simulink model "Zone_1_Zone_2_Thyristor_240Hz"  (R2025b)
settings: Solver=FixedStepDiscrete  StartTime=0.0  StopTime=5  FixedStep=Ts  RelTol=1e-3  EnableMultiTasking=on
undefined symbols (not defined in the file or in its folder): DiscIntNeverNeededParam, GABDA, GABDB, GBBDA, GBBDB, GPPMA, GPPMB, GPPMC, SADA, SADB, SADC, SADD, SBDA, SBDB, SBDC, SCDA, SCDB, SCDC, SCDD, SDDA, SDDB, SDDC, SDDD, SDDE, Ts, TsELEC
libraries: nesl_utility x70, fl_lib x60, ee_lib x44, eeThyristorSixPulseGenerator x2, eePowerMeasurement x2, eeSinusoidalMeasurement x2
(part 1 of 3)
settings Model: Creator=gdudgeon  LastModifiedBy=gdudgeon
settings SolverCC: ConcurrentTasks=on  AlgebraicLoopSolver=TrustRegion  AutoInsertRateTranBlk=on
settings DataIOCC: SaveFormat=StructureWithTime  SaveOutput=off  SignalLogging=off  DSMLogging=off  SaveTime=off
settings OptimizationCC: BlockReduction=off  OptimizeBlockIOStorage=off  BufferReuse=off  GlobalBufferReuse=off  ExpressionFolding=off  LocalBlockOutputs=off  OptimizeDataStoreBuffers=off  BusAssignmentInplaceUpdate=off
settings DebuggingCC: UnconnectedInputMsg=warning  UnconnectedOutputMsg=warning  UnconnectedLineMsg=warning
settings HardwareCC: ProdBitPerPointer=32.0  ProdBitPerSizeT=32.0  ProdBitPerPtrDiffT=32.0  ProdLargestAtomicFloat=None  ProdWordSize=32.0  ProdLongLongMode=on  ProdHWDeviceType=Generic->32-bit x86 compatible
settings ModelReferenceCC: EnableRefExpFcnMdlSchedulingChecks=on  ModelReferenceNumInstancesAllowed=Single  ModelReferenceMinAlgLoopOccurrences=on
settings SFSimCC: CustomCodeUndefinedFunction=UseInterfaceOnly
settings RTWCC: SystemTargetFile=slrt.tlc  TLCOptions=-axPCMaxOverloads=3000  TemplateMakefile=slrt_default_tmf  CodeProfilingInstrumentation=coarse  RTWCompilerOptimization=on  GPUComputeCapability=3.5  Description=Simulink Real-Time
settings SimulinkRealTimeCC: RL32LogTETModifier=off  xPCConcurrentTasks=on  MultiwordLength=2048.0  DynamicStringBufferSize=256.0  PreserveMATLABNamespacesInGeneratedCode=on  SubcomponentCodeInterfacePackaging=Nonreusable function  SupportVariableSizeSignals=on  InstructionSetFMA=off  OptimizeReductions=off  LogToMDFFile=off

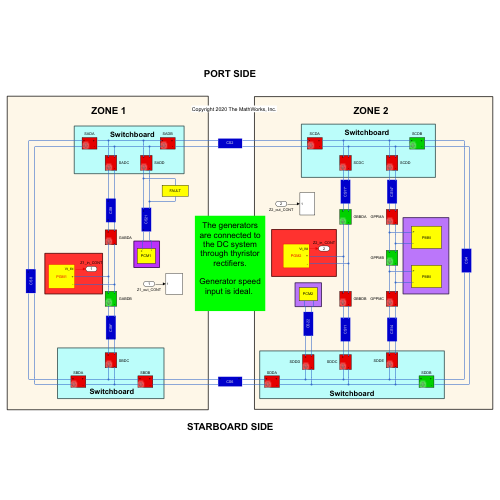
[thumbnail: Simulink's stored preview of the top-level diagram]
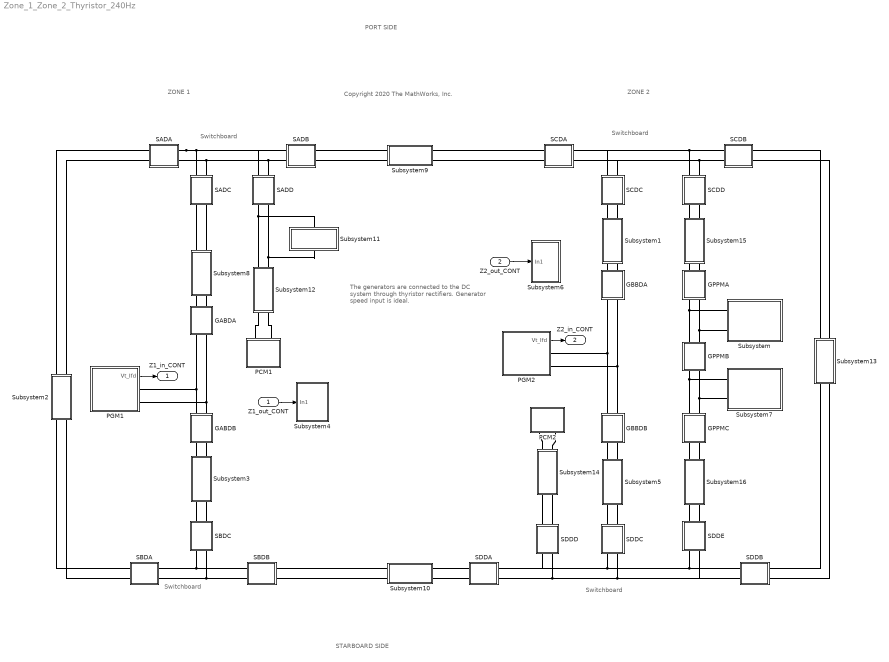
== system Zone_1_Zone_2_Thyristor_240Hz ==
  note: Copyright 2020 The MathWorks, Inc.
  note: The generators are connected to the DC system through thyristor rectifiers.
      |
      | Generator speed input is ideal.
  note: Switchboard
  note: Switchboard
  note: Switchboard
  note: ZONE 1
  note: Switchboard
  note: ZONE 2
  note: PORT SIDE
  note: STARBOARD SIDE
  Z1_out_CONT : Inport  OutDataTypeStr=double  PortDimensions=11
  Z2_out_CONT : Inport  Port=2  OutDataTypeStr=double  PortDimensions=17
  GABDA : Subsystem  mask{status=GABDA}
      mask prompts: status "Initial Status"
      mask init:
      | if ~status
      |     
      |     set(gcbh,'BackgroundColor','green')
      |     
      | elseif status
      |     
      |     set(gcbh,'BackgroundColor','red')
      |     
      | end
  GABDB : Subsystem  mask{status=GABDB}
      mask prompts: status "Initial Status"
      mask init:
      | if ~status
      |     
      |     set(gcbh,'BackgroundColor','green')
      |     
      | elseif status
      |     
      |     set(gcbh,'BackgroundColor','red')
      |     
      | end
  GBBDA : Subsystem  mask{status=GBBDA}
      mask prompts: status "Initial Status"
      mask init:
      | if ~status
      |     
      |     set(gcbh,'BackgroundColor','green')
      |     
      | elseif status
      |     
      |     set(gcbh,'BackgroundColor','red')
      |     
      | end
  GBBDB : Subsystem  mask{status=GBBDB}
      mask prompts: status "Initial Status"
      mask init:
      | if ~status
      |     
      |     set(gcbh,'BackgroundColor','green')
      |     
      | elseif status
      |     
      |     set(gcbh,'BackgroundColor','red')
      |     
      | end
  GPPMA : Subsystem  mask{status=GPPMA}
      mask prompts: status "Initial Status"
      mask init:
      | if ~status
      |     
      |     set(gcbh,'BackgroundColor','green')
      |     
      | elseif status
      |     
      |     set(gcbh,'BackgroundColor','red')
      |     
      | end
  GPPMB : Subsystem  mask{status=GPPMB}
      mask prompts: status "Initial Status"
      mask init:
      | if ~status
      |     
      |     set(gcbh,'BackgroundColor','green')
      |     
      | elseif status
      |     
      |     set(gcbh,'BackgroundColor','red')
      |     
      | end
  GPPMC : Subsystem  mask{status=GPPMC}
      mask prompts: status "Initial Status"
      mask init:
      | if ~status
      |     
      |     set(gcbh,'BackgroundColor','green')
      |     
      | elseif status
      |     
      |     set(gcbh,'BackgroundColor','red')
      |     
      | end
  PCM1 : Subsystem
      mask Display: disp('PCM1')
  PCM2 : Subsystem
      mask Display: disp('PCM2')
  PGM1 : Subsystem
      mask Display: disp('PGM1')
  PGM2 : Subsystem
      mask Display: disp('PGM2')
  SADA : Subsystem  mask{status=SADA}
      mask prompts: status "Initial Status"
      mask init:
      | if ~status
      |     
      |     set(gcbh,'BackgroundColor','green')
      |     
      | elseif status
      |     
      |     set(gcbh,'BackgroundColor','red')
      |     
      | end
  SADB : Subsystem  mask{status=SADB}
      mask prompts: status "Initial Status"
      mask init:
      | if ~status
      |     
      |     set(gcbh,'BackgroundColor','green')
      |     
      | elseif status
      |     
      |     set(gcbh,'BackgroundColor','red')
      |     
      | end
  SADC : Subsystem  mask{status=SADC}
      mask prompts: status "Initial Status"
      mask init:
      | if ~status
      |     
      |     set(gcbh,'BackgroundColor','green')
      |     
      | elseif status
      |     
      |     set(gcbh,'BackgroundColor','red')
      |     
      | end
  SADD : Subsystem  mask{status=SADD}
      mask prompts: status "Initial Status"
      mask init:
      | if ~status
      |     
      |     set(gcbh,'BackgroundColor','green')
      |     
      | elseif status
      |     
      |     set(gcbh,'BackgroundColor','red')
      |     
      | end
  SBDA : Subsystem  mask{status=SBDA}
      mask prompts: status "Initial Status"
      mask init:
      | if ~status
      |     
      |     set(gcbh,'BackgroundColor','green')
      |     
      | elseif status
      |     
      |     set(gcbh,'BackgroundColor','red')
      |     
      | end
  SBDB : Subsystem  mask{status=SBDB}
      mask prompts: status "Initial Status"
      mask init:
      | if ~status
      |     
      |     set(gcbh,'BackgroundColor','green')
      |     
      | elseif status
      |     
      |     set(gcbh,'BackgroundColor','red')
      |     
      | end
  SBDC : Subsystem  mask{status=SBDC}
      mask prompts: status "Initial Status"
      mask init:
      | if ~status
      |     
      |     set(gcbh,'BackgroundColor','green')
      |     
      | elseif status
      |     
      |     set(gcbh,'BackgroundColor','red')
      |     
      | end
  SCDA : Subsystem  mask{status=SCDA}
      mask prompts: status "Initial Status"
      mask init:
      | if ~status
      |     
      |     set(gcbh,'BackgroundColor','green')
      |     
      | elseif status
      |     
      |     set(gcbh,'BackgroundColor','red')
      |     
      | end
  SCDB : Subsystem  mask{status=SCDB}
      mask prompts: status "Initial Status"
      mask init:
      | if ~status
      |     
      |     set(gcbh,'BackgroundColor','green')
      |     
      | elseif status
      |     
      |     set(gcbh,'BackgroundColor','red')
      |     
      | end
  SCDC : Subsystem  mask{status=SCDC}
      mask prompts: status "Initial Status"
      mask init:
      | if ~status
      |     
      |     set(gcbh,'BackgroundColor','green')
      |     
      | elseif status
      |     
      |     set(gcbh,'BackgroundColor','red')
      |     
      | end
  SCDD : Subsystem  mask{status=SCDD}
      mask prompts: status "Initial Status"
      mask init:
      | if ~status
      |     
      |     set(gcbh,'BackgroundColor','green')
      |     
      | elseif status
      |     
      |     set(gcbh,'BackgroundColor','red')
      |     
      | end
  SDDA : Subsystem  mask{status=SDDA}
      mask prompts: status "Initial Status"
      mask init:
      | if ~status
      |     
      |     set(gcbh,'BackgroundColor','green')
      |     
      | elseif status
      |     
      |     set(gcbh,'BackgroundColor','red')
      |     
      | end
  SDDB : Subsystem  mask{status=SDDB}
      mask prompts: status "Initial Status"
      mask init:
      | if ~status
      |     
      |     set(gcbh,'BackgroundColor','green')
      |     
      | elseif status
      |     
      |     set(gcbh,'BackgroundColor','red')
      |     
      | end
  SDDC : Subsystem  mask{status=SDDC}
      mask prompts: status "Initial Status"
      mask init:
      | if ~status
      |     
      |     set(gcbh,'BackgroundColor','green')
      |     
      | elseif status
      |     
      |     set(gcbh,'BackgroundColor','red')
      |     
      | end
  SDDD : Subsystem  mask{status=SDDD}
      mask prompts: status "Initial Status"
      mask init:
      | if ~status
      |     
      |     set(gcbh,'BackgroundColor','green')
      |     
      | elseif status
      |     
      |     set(gcbh,'BackgroundColor','red')
      |     
      | end
  SDDE : Subsystem  mask{status=SDDE}
      mask prompts: status "Initial Status"
      mask init:
      | if ~status
      |     
      |     set(gcbh,'BackgroundColor','green')
      |     
      | elseif status
      |     
      |     set(gcbh,'BackgroundColor','red')
      |     
      | end
  Subsystem : Subsystem
      mask Display: disp('PMM')
  Subsystem1 : Subsystem
      mask Display: disp('CS11*')
  Subsystem10 : Subsystem
      mask Display: disp('CS6')
  Subsystem11 : Subsystem
      mask Display: disp('FAULT')
  Subsystem12 : Subsystem
      mask Display: disp('CS21')
  Subsystem13 : Subsystem
      mask Display: disp('CS4')
  Subsystem14 : Subsystem
      mask Display: disp('CS22')
  Subsystem15 : Subsystem
      mask Display: disp('CS14*')
  Subsystem16 : Subsystem
      mask Display: disp('CS14')
  Subsystem2 : Subsystem
      mask Display: disp('CS8')
  Subsystem3 : Subsystem
      mask Display: disp('CS9*')
  Subsystem4 : Subsystem
  Subsystem5 : Subsystem
      mask Display: disp('CS11')
  Subsystem6 : Subsystem
  Subsystem7 : Subsystem
      mask Display: disp('PMM')
  Subsystem8 : Subsystem
      mask Display: disp('CS9')
  Subsystem9 : Subsystem
      mask Display: disp('CS2')
  Z1_in_CONT : Outport  OutDataTypeStr=double  PortDimensions=2
  Z2_in_CONT : Outport  Port=2  OutDataTypeStr=double  PortDimensions=2
  wires:
  PGM2/1(Vt_Ifd) -> Z2_in_CONT/1
  PGM1/1(Vt_Ifd) -> Z1_in_CONT/1
  Z1_out_CONT/1 -> Subsystem4/1(In1)
  Z2_out_CONT/1 -> Subsystem6/1(In1)
  connections:
  GBBDA/RConn1 -- PGM2/RConn1 -- GBBDB/LConn1
  SDDB/LConn2 -- SDDE/RConn2 -- SDDC/RConn2 -- SDDD/RConn2 -- SDDA/RConn2
  SDDD/RConn1 -- SDDA/RConn1 -- SDDC/RConn1 -- SDDB/LConn1 -- SDDE/RConn1
  GBBDB/LConn2 -- PGM2/RConn2 -- GBBDA/RConn2
  Subsystem16/RConn2 -- SDDE/LConn2
  GBBDB/RConn1 -- Subsystem5/LConn1
  Subsystem16/RConn1 -- SDDE/LConn1
  SDDC/LConn1 -- Subsystem5/RConn1
  SDDC/LConn2 -- Subsystem5/RConn2
  Subsystem10/LConn1 -- SDDA/LConn1
  GBBDB/RConn2 -- Subsystem5/LConn2
  Subsystem10/LConn2 -- SDDA/LConn2
  SCDD/LConn2 -- SCDB/LConn2 -- SCDA/RConn2 -- SCDC/LConn2
  SCDD/LConn1 -- SCDB/LConn1 -- SCDA/RConn1 -- SCDC/LConn1
  Subsystem15/LConn1 -- SCDD/RConn1
  Subsystem15/LConn2 -- SCDD/RConn2
  GBBDA/LConn2 -- Subsystem1/RConn2
  GBBDA/LConn1 -- Subsystem1/RConn1
  SCDC/RConn1 -- Subsystem1/LConn1
  SCDC/RConn2 -- Subsystem1/LConn2
  Subsystem13/LConn1 -- SCDB/RConn1
  SCDB/RConn2 -- Subsystem13/LConn2
  Subsystem13/RConn1 -- SDDB/RConn1
  SDDB/RConn2 -- Subsystem13/RConn2
  SADA/RConn2 -- SADB/LConn2 -- SADD/LConn2 -- SADC/LConn2
  SBDC/RConn2 -- SBDA/RConn2 -- SBDB/LConn2
  GABDB/LConn2 -- PGM1/RConn2 -- GABDA/RConn2
  GABDB/LConn1 -- PGM1/RConn1 -- GABDA/RConn1
  SADA/RConn1 -- SADC/LConn1 -- SADB/LConn1 -- SADD/LConn1
  SBDC/RConn1 -- SBDA/RConn1 -- SBDB/LConn1
  GABDB/RConn1 -- Subsystem3/LConn1
  GABDA/LConn2 -- Subsystem8/RConn2
  GABDA/LConn1 -- Subsystem8/RConn1
  SBDA/LConn1 -- Subsystem2/RConn1
  Subsystem2/LConn2 -- SADA/LConn2
  SADC/RConn2 -- Subsystem8/LConn2
  SADC/RConn1 -- Subsystem8/LConn1
  Subsystem10/RConn2 -- SBDB/RConn2
  Subsystem2/LConn1 -- SADA/LConn1
  GABDB/RConn2 -- Subsystem3/LConn2
  SBDC/LConn2 -- Subsystem3/RConn2
  Subsystem10/RConn1 -- SBDB/RConn1
  SBDC/LConn1 -- Subsystem3/RConn1
  SBDA/LConn2 -- Subsystem2/RConn2
  Subsystem9/RConn1 -- SADB/RConn1
  Subsystem9/RConn2 -- SADB/RConn2
  SCDA/LConn1 -- Subsystem9/LConn1
  Subsystem9/LConn2 -- SCDA/LConn2
  Subsystem12/RConn2 -- PCM1/LConn2
  Subsystem12/RConn1 -- PCM1/LConn1
  Subsystem12/LConn1 -- Subsystem11/LConn1 -- SADD/RConn1
  SADD/RConn2 -- Subsystem11/RConn1 -- Subsystem12/LConn2
  Subsystem14/LConn1 -- PCM2/LConn1
  PCM2/LConn2 -- Subsystem14/LConn2
  Subsystem14/RConn1 -- SDDD/LConn1
  SDDD/LConn2 -- Subsystem14/RConn2
  GPPMC/RConn2 -- Subsystem16/LConn2
  GPPMC/RConn1 -- Subsystem16/LConn1
  GPPMA/LConn1 -- Subsystem15/RConn1
  GPPMA/LConn2 -- Subsystem15/RConn2
  GPPMA/RConn1 -- Subsystem/LConn1 -- GPPMB/LConn1
  GPPMA/RConn2 -- Subsystem/LConn2 -- GPPMB/LConn2
  GPPMB/RConn1 -- Subsystem7/LConn1 -- GPPMC/LConn1
  GPPMB/RConn2 -- Subsystem7/LConn2 -- GPPMC/LConn2

== system Zone_1_Zone_2_Thyristor_240Hz/GABDA ==
  SADC : ee_lib/Switches & Breakers/DPST Switch  R_closed=1e-3 Ohm  G_open=1e-6 S  Threshold=0.5 V  Width=0 V  model_dynamics=0  t_on=1e-3 s  t_off=1e-3 s  initial_vT=0 V
      settings: InternalSimscapePortConfiguration="{\"Bottom\":[],\"Left\":[{\"id\":\"vT\",\"label\":\"vT\",\"type\":\"input\"},{\"id\":\"p1\",\"label\":\"\",\"type\":\"foundation.electrical.electrical\"},{\"id\":\"p2\",\"label\":\"\",\"type\":\"foundation.electrical.electrical\"}],\"Right\":[{\"id\":\"n1\",\"label\":\"\",\"type\":\"foundation.electrical.electrical\"},{\"id\":\"n2\",\"label\":\"\",\"type\":\"foundation.electrical.electrical\"}],\"Top\":[]}"
  Simulink-PS Converter : nesl_utility/Simulink-PS Converter  PhysicalDomain=network_engine_domain  SubClassName=ps_input  LeftPortType=input  RightPortType=output  PseudoPeriodic=off  Frequencies=[]  NoiseDistribution=none  NoiseParameters=[]  Unit=1  AffineConversion=off  FilteringAndDerivatives=provide  SimscapeFilterOrder=1  InputFilterTimeConstant=0.001  UdotUserProvided=0
  "+ " : PMIOPort  Side=Right
  + : PMIOPort  Port=2  Side=Left
  "- " : PMIOPort  Port=3  Side=Right
  - : PMIOPort  Port=4  Side=Left
  wires:
  [GABDA] -> Simulink-PS Converter/1  "GABDA"
  connections:
  Simulink-PS Converter/RConn1 -- SADC/LConn1
  SADC/LConn2 -- +/RConn1
  SADC/LConn3 -- -/RConn1
  SADC/RConn2 -- "- "/RConn1
  SADC/RConn1 -- "+ "/RConn1

== system Zone_1_Zone_2_Thyristor_240Hz/GABDB ==
  GABDB : ee_lib/Switches & Breakers/DPST Switch  R_closed=1e-3 Ohm  G_open=1e-6 S  Threshold=0.5 V  Width=0 V  model_dynamics=0  t_on=1e-3 s  t_off=1e-3 s  initial_vT=0 V
      settings: InternalSimscapePortConfiguration="{\"Bottom\":[],\"Left\":[{\"id\":\"vT\",\"label\":\"vT\",\"type\":\"input\"},{\"id\":\"p1\",\"label\":\"\",\"type\":\"foundation.electrical.electrical\"},{\"id\":\"p2\",\"label\":\"\",\"type\":\"foundation.electrical.electrical\"}],\"Right\":[{\"id\":\"n1\",\"label\":\"\",\"type\":\"foundation.electrical.electrical\"},{\"id\":\"n2\",\"label\":\"\",\"type\":\"foundation.electrical.electrical\"}],\"Top\":[]}"
  Simulink-PS Converter : nesl_utility/Simulink-PS Converter  PhysicalDomain=network_engine_domain  SubClassName=ps_input  LeftPortType=input  RightPortType=output  PseudoPeriodic=off  Frequencies=[]  NoiseDistribution=none  NoiseParameters=[]  Unit=1  AffineConversion=off  FilteringAndDerivatives=provide  SimscapeFilterOrder=1  InputFilterTimeConstant=0.001  UdotUserProvided=0
  "+ " : PMIOPort  Side=Right
  + : PMIOPort  Port=2  Side=Left
  "- " : PMIOPort  Port=3  Side=Right
  - : PMIOPort  Port=4  Side=Left
  wires:
  [GABDB] -> Simulink-PS Converter/1
  connections:
  GABDB/RConn1 -- "+ "/RConn1
  GABDB/LConn3 -- -/RConn1
  GABDB/RConn2 -- "- "/RConn1
  Simulink-PS Converter/RConn1 -- GABDB/LConn1
  GABDB/LConn2 -- +/RConn1

== system Zone_1_Zone_2_Thyristor_240Hz/GBBDA ==
  SADC : ee_lib/Switches & Breakers/DPST Switch  R_closed=1e-3 Ohm  G_open=1e-6 S  Threshold=0.5 V  Width=0 V  model_dynamics=0  t_on=1e-3 s  t_off=1e-3 s  initial_vT=0 V
      settings: InternalSimscapePortConfiguration="{\"Bottom\":[],\"Left\":[{\"id\":\"vT\",\"label\":\"vT\",\"type\":\"input\"},{\"id\":\"p1\",\"label\":\"\",\"type\":\"foundation.electrical.electrical\"},{\"id\":\"p2\",\"label\":\"\",\"type\":\"foundation.electrical.electrical\"}],\"Right\":[{\"id\":\"n1\",\"label\":\"\",\"type\":\"foundation.electrical.electrical\"},{\"id\":\"n2\",\"label\":\"\",\"type\":\"foundation.electrical.electrical\"}],\"Top\":[]}"
  Simulink-PS Converter : nesl_utility/Simulink-PS Converter  PhysicalDomain=network_engine_domain  SubClassName=ps_input  LeftPortType=input  RightPortType=output  PseudoPeriodic=off  Frequencies=[]  NoiseDistribution=none  NoiseParameters=[]  Unit=1  AffineConversion=off  FilteringAndDerivatives=provide  SimscapeFilterOrder=1  InputFilterTimeConstant=0.001  UdotUserProvided=0
  "+ " : PMIOPort  Side=Right
  + : PMIOPort  Port=2  Side=Left
  "- " : PMIOPort  Port=3  Side=Right
  - : PMIOPort  Port=4  Side=Left
  wires:
  [GBBDA] -> Simulink-PS Converter/1
  connections:
  SADC/LConn1 -- Simulink-PS Converter/RConn1
  SADC/RConn1 -- "+ "/RConn1
  SADC/RConn2 -- "- "/RConn1
  SADC/LConn2 -- +/RConn1
  SADC/LConn3 -- -/RConn1

== system Zone_1_Zone_2_Thyristor_240Hz/GBBDB ==
  GBBDB : ee_lib/Switches & Breakers/DPST Switch  R_closed=1e-3 Ohm  G_open=1e-6 S  Threshold=0.5 V  Width=0 V  model_dynamics=0  t_on=1e-3 s  t_off=1e-3 s  initial_vT=0 V
      settings: InternalSimscapePortConfiguration="{\"Bottom\":[],\"Left\":[{\"id\":\"vT\",\"label\":\"vT\",\"type\":\"input\"},{\"id\":\"p1\",\"label\":\"\",\"type\":\"foundation.electrical.electrical\"},{\"id\":\"p2\",\"label\":\"\",\"type\":\"foundation.electrical.electrical\"}],\"Right\":[{\"id\":\"n1\",\"label\":\"\",\"type\":\"foundation.electrical.electrical\"},{\"id\":\"n2\",\"label\":\"\",\"type\":\"foundation.electrical.electrical\"}],\"Top\":[]}"
  Simulink-PS Converter : nesl_utility/Simulink-PS Converter  PhysicalDomain=network_engine_domain  SubClassName=ps_input  LeftPortType=input  RightPortType=output  PseudoPeriodic=off  Frequencies=[]  NoiseDistribution=none  NoiseParameters=[]  Unit=1  AffineConversion=off  FilteringAndDerivatives=provide  SimscapeFilterOrder=1  InputFilterTimeConstant=0.001  UdotUserProvided=0
  "+ " : PMIOPort  Side=Right
  + : PMIOPort  Port=2  Side=Left
  "- " : PMIOPort  Port=3  Side=Right
  - : PMIOPort  Port=4  Side=Left
  wires:
  [GBBDB] -> Simulink-PS Converter/1
  connections:
  GBBDB/RConn1 -- "+ "/RConn1
  GBBDB/LConn3 -- -/RConn1
  GBBDB/RConn2 -- "- "/RConn1
  Simulink-PS Converter/RConn1 -- GBBDB/LConn1
  GBBDB/LConn2 -- +/RConn1

== system Zone_1_Zone_2_Thyristor_240Hz/GPPMA ==
  SADC : ee_lib/Switches & Breakers/DPST Switch  R_closed=1e-3 Ohm  G_open=1e-6 S  Threshold=0.5 V  Width=0 V  model_dynamics=0  t_on=1e-3 s  t_off=1e-3 s  initial_vT=0 V
      settings: InternalSimscapePortConfiguration="{\"Bottom\":[],\"Left\":[{\"id\":\"vT\",\"label\":\"vT\",\"type\":\"input\"},{\"id\":\"p1\",\"label\":\"\",\"type\":\"foundation.electrical.electrical\"},{\"id\":\"p2\",\"label\":\"\",\"type\":\"foundation.electrical.electrical\"}],\"Right\":[{\"id\":\"n1\",\"label\":\"\",\"type\":\"foundation.electrical.electrical\"},{\"id\":\"n2\",\"label\":\"\",\"type\":\"foundation.electrical.electrical\"}],\"Top\":[]}"
  Simulink-PS Converter : nesl_utility/Simulink-PS Converter  PhysicalDomain=network_engine_domain  SubClassName=ps_input  LeftPortType=input  RightPortType=output  PseudoPeriodic=off  Frequencies=[]  NoiseDistribution=none  NoiseParameters=[]  Unit=1  AffineConversion=off  FilteringAndDerivatives=provide  SimscapeFilterOrder=1  InputFilterTimeConstant=0.001  UdotUserProvided=0
  "+ " : PMIOPort  Side=Right
  + : PMIOPort  Port=2  Side=Left
  "- " : PMIOPort  Port=3  Side=Right
  - : PMIOPort  Port=4  Side=Left
  wires:
  [GPPMA] -> Simulink-PS Converter/1
  connections:
  SADC/RConn2 -- "- "/RConn1
  SADC/RConn1 -- "+ "/RConn1
  SADC/LConn2 -- +/RConn1
  SADC/LConn3 -- -/RConn1
  Simulink-PS Converter/RConn1 -- SADC/LConn1

== system Zone_1_Zone_2_Thyristor_240Hz/GPPMB ==
  SADC : ee_lib/Switches & Breakers/DPST Switch  R_closed=1e-3 Ohm  G_open=1e-6 S  Threshold=0.5 V  Width=0 V  model_dynamics=0  t_on=1e-3 s  t_off=1e-3 s  initial_vT=0 V
      settings: InternalSimscapePortConfiguration="{\"Bottom\":[],\"Left\":[{\"id\":\"vT\",\"label\":\"vT\",\"type\":\"input\"},{\"id\":\"p1\",\"label\":\"\",\"type\":\"foundation.electrical.electrical\"},{\"id\":\"p2\",\"label\":\"\",\"type\":\"foundation.electrical.electrical\"}],\"Right\":[{\"id\":\"n1\",\"label\":\"\",\"type\":\"foundation.electrical.electrical\"},{\"id\":\"n2\",\"label\":\"\",\"type\":\"foundation.electrical.electrical\"}],\"Top\":[]}"
  Simulink-PS Converter : nesl_utility/Simulink-PS Converter  PhysicalDomain=network_engine_domain  SubClassName=ps_input  LeftPortType=input  RightPortType=output  PseudoPeriodic=off  Frequencies=[]  NoiseDistribution=none  NoiseParameters=[]  Unit=1  AffineConversion=off  FilteringAndDerivatives=provide  SimscapeFilterOrder=1  InputFilterTimeConstant=0.001  UdotUserProvided=0
  "+ " : PMIOPort  Side=Right
  + : PMIOPort  Port=2  Side=Left
  "- " : PMIOPort  Port=3  Side=Right
  - : PMIOPort  Port=4  Side=Left
  wires:
  [GPPMB] -> Simulink-PS Converter/1
  connections:
  Simulink-PS Converter/RConn1 -- SADC/LConn1
  SADC/LConn3 -- -/RConn1
  SADC/LConn2 -- +/RConn1
  SADC/RConn1 -- "+ "/RConn1
  SADC/RConn2 -- "- "/RConn1

== system Zone_1_Zone_2_Thyristor_240Hz/GPPMC ==
  SADC : ee_lib/Switches & Breakers/DPST Switch  R_closed=1e-3 Ohm  G_open=1e-6 S  Threshold=0.5 V  Width=0 V  model_dynamics=0  t_on=1e-3 s  t_off=1e-3 s  initial_vT=0 V
      settings: InternalSimscapePortConfiguration="{\"Bottom\":[],\"Left\":[{\"id\":\"vT\",\"label\":\"vT\",\"type\":\"input\"},{\"id\":\"p1\",\"label\":\"\",\"type\":\"foundation.electrical.electrical\"},{\"id\":\"p2\",\"label\":\"\",\"type\":\"foundation.electrical.electrical\"}],\"Right\":[{\"id\":\"n1\",\"label\":\"\",\"type\":\"foundation.electrical.electrical\"},{\"id\":\"n2\",\"label\":\"\",\"type\":\"foundation.electrical.electrical\"}],\"Top\":[]}"
  Simulink-PS Converter : nesl_utility/Simulink-PS Converter  PhysicalDomain=network_engine_domain  SubClassName=ps_input  LeftPortType=input  RightPortType=output  PseudoPeriodic=off  Frequencies=[]  NoiseDistribution=none  NoiseParameters=[]  Unit=1  AffineConversion=off  FilteringAndDerivatives=provide  SimscapeFilterOrder=1  InputFilterTimeConstant=0.001  UdotUserProvided=0
  "+ " : PMIOPort  Side=Right
  + : PMIOPort  Port=2  Side=Left
  "- " : PMIOPort  Port=3  Side=Right
  - : PMIOPort  Port=4  Side=Left
  wires:
  [GPPMC] -> Simulink-PS Converter/1
  connections:
  SADC/RConn2 -- "- "/RConn1
  SADC/RConn1 -- "+ "/RConn1
  SADC/LConn2 -- +/RConn1
  SADC/LConn3 -- -/RConn1
  Simulink-PS Converter/RConn1 -- SADC/LConn1

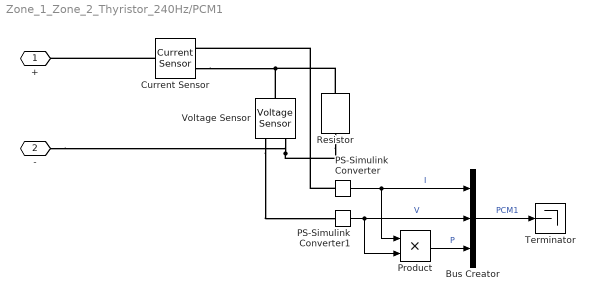
== system Zone_1_Zone_2_Thyristor_240Hz/PCM1 ==
  Bus Creator : BusCreator  Inputs=3
  Current Sensor : fl_lib/Electrical/Electrical Sensors/Current Sensor
  PS-Simulink Converter : nesl_utility/PS-Simulink Converter  PhysicalDomain=network_engine_domain  SubClassName=ps_output  LeftPortType=input  RightPortType=output  PseudoPeriodic=off  Frequencies=[]  VectorFormat=1-D array  Unit=1  AffineConversion=off
  PS-Simulink Converter1 : nesl_utility/PS-Simulink Converter  PhysicalDomain=network_engine_domain  SubClassName=ps_output  LeftPortType=input  RightPortType=output  PseudoPeriodic=off  Frequencies=[]  VectorFormat=1-D array  Unit=1  AffineConversion=off
  Product : Product
  Resistor : fl_lib/Electrical/Electrical Elements/Resistor  R=20 Ohm  i_specify=off  i_priority=None  i=0 A  i_nominal_specify=off  i_nominal_value=1  i_nominal_unit=A  v_specify=off  v_priority=None  v=0 V  v_nominal_specify=off  v_nominal_value=1  v_nominal_unit=V
  Terminator : Terminator
  Voltage Sensor : fl_lib/Electrical/Electrical Sensors/Voltage Sensor
  + : PMIOPort  Side=Left
  - : PMIOPort  Port=2  Side=Left
  wires:
  PS-Simulink Converter/1 -> Product/1, Bus Creator/1  "I"
  PS-Simulink Converter1/1 -> Product/2, Bus Creator/2  "V"
  Product/1 -> Bus Creator/3  "P"
  Bus Creator/1 -> Terminator/1  "PCM1"
  connections:
  Current Sensor/RConn2 -- Resistor/LConn1 -- Voltage Sensor/LConn1
  Voltage Sensor/RConn2 -- -/RConn1 -- Resistor/RConn1
  PS-Simulink Converter/LConn1 -- Current Sensor/RConn1
  Voltage Sensor/RConn1 -- PS-Simulink Converter1/LConn1
  Current Sensor/LConn1 -- +/RConn1

== system Zone_1_Zone_2_Thyristor_240Hz/PCM2 ==
  Bus Creator : BusCreator  Inputs=3
  Current Sensor : fl_lib/Electrical/Electrical Sensors/Current Sensor
  PS-Simulink Converter : nesl_utility/PS-Simulink Converter  PhysicalDomain=network_engine_domain  SubClassName=ps_output  LeftPortType=input  RightPortType=output  PseudoPeriodic=off  Frequencies=[]  VectorFormat=1-D array  Unit=1  AffineConversion=off
  PS-Simulink Converter1 : nesl_utility/PS-Simulink Converter  PhysicalDomain=network_engine_domain  SubClassName=ps_output  LeftPortType=input  RightPortType=output  PseudoPeriodic=off  Frequencies=[]  VectorFormat=1-D array  Unit=1  AffineConversion=off
  Product : Product
  Resistor : fl_lib/Electrical/Electrical Elements/Resistor  R=100 Ohm  i_specify=off  i_priority=None  i=0 A  i_nominal_specify=off  i_nominal_value=1  i_nominal_unit=A  v_specify=off  v_priority=None  v=0 V  v_nominal_specify=off  v_nominal_value=1  v_nominal_unit=V
  Terminator : Terminator
  Voltage Sensor : fl_lib/Electrical/Electrical Sensors/Voltage Sensor
  + : PMIOPort  Side=Left
  - : PMIOPort  Port=2  Side=Left
  wires:
  PS-Simulink Converter/1 -> Product/1, Bus Creator/1  "I"
  PS-Simulink Converter1/1 -> Product/2, Bus Creator/2  "V"
  Product/1 -> Bus Creator/3  "P"
  Bus Creator/1 -> Terminator/1  "PCM2"
  connections:
  Current Sensor/RConn2 -- Resistor/LConn1 -- Voltage Sensor/LConn1
  Voltage Sensor/RConn2 -- -/RConn1 -- Resistor/RConn1
  PS-Simulink Converter/LConn1 -- Current Sensor/RConn1
  Voltage Sensor/RConn1 -- PS-Simulink Converter1/LConn1
  +/RConn1 -- Current Sensor/LConn1

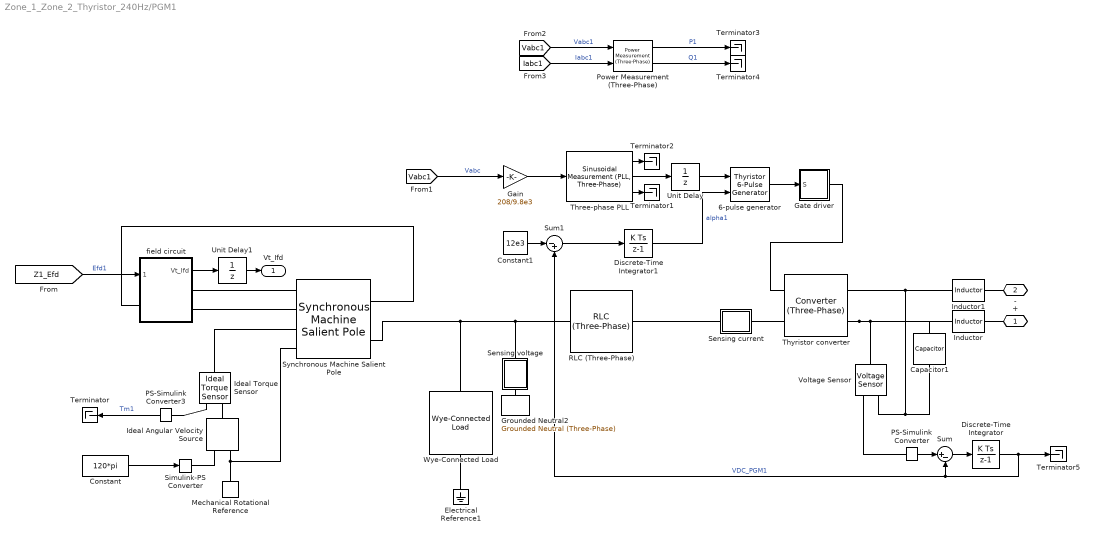
== system Zone_1_Zone_2_Thyristor_240Hz/PGM1 ==
  " field circuit" : Subsystem
  6-pulse generator : eeThyristorSixPulseGenerator/Thyristor 6-Pulse Generator  Ord=Sequential device order  Pw=5*pi/6  Ts=TsELEC
  Capacitor1 : fl_lib/Electrical/Electrical Elements/Capacitor  c=835e-6 F  r=0.075 Ohm  g=0 1/Ohm  i_specify=off  i_priority=None  i=0 A  i_nominal_specify=off  i_nominal_value=1  i_nominal_unit=A  v_specify=on  v_priority=None  v=12e3 V  v_nominal_specify=off  v_nominal_value=1  v_nominal_unit=V  vc_specify=on  vc_priority=High  vc=12e3 V  vc_nominal_specify=off  vc_nominal_value=1  vc_nominal_unit=V
  Constant : Constant  Value=120*pi  SampleTime=TsELEC
  Constant1 : Constant  Value=12e3
  Discrete-Time Integrator : DiscreteIntegrator  gainval=100  InitialCondition=12e3  SampleTime=TsELEC  ICPrevOutput=DiscIntNeverNeededParam  ICPrevScaledInput=DiscIntNeverNeededParam
  Discrete-Time Integrator1 : DiscreteIntegrator  gainval=0.01  InitialCondition=0.9  SampleTime=TsELEC  LimitOutput=on  LowerSaturationLimit=0  ICPrevOutput=DiscIntNeverNeededParam  ICPrevScaledInput=DiscIntNeverNeededParam
  Electrical Reference1 : fl_lib/Electrical/Electrical Elements/Electrical Reference
  Gain : Gain  Gain=208/9.8e3
  Gate driver : Subsystem
  Grounded Neutral2 : ee_lib/Connectors & References/Grounded Neutral (Three-Phase)
  Ideal Angular Velocity Source : fl_lib/Mechanical/Mechanical Sources/Ideal Angular Velocity Source
  Ideal Torque Sensor : fl_lib/Mechanical/Mechanical Sensors/Ideal Torque Sensor
  Inductor : fl_lib/Electrical/Electrical Elements/Inductor  l=790e-6/2 H  r=0.075/2 Ohm  g=1e-9 1/Ohm  i_specify=off  i_priority=None  i=0 A  i_nominal_specify=off  i_nominal_value=1  i_nominal_unit=A  v_specify=off  v_priority=None  v=0 V  v_nominal_specify=off  v_nominal_value=1  v_nominal_unit=V  i_L_specify=off  i_L_priority=High  i_L=0 A  i_L_nominal_specify=off  i_L_nominal_value=1  i_L_nominal_unit=A
  Inductor1 : fl_lib/Electrical/Electrical Elements/Inductor  l=790e-6/2 H  r=0.075/2 Ohm  g=1e-9 1/Ohm  i_specify=off  i_priority=None  i=0 A  i_nominal_specify=off  i_nominal_value=1  i_nominal_unit=A  v_specify=off  v_priority=None  v=0 V  v_nominal_specify=off  v_nominal_value=1  v_nominal_unit=V  i_L_specify=off  i_L_priority=High  i_L=0 A  i_L_nominal_specify=off  i_L_nominal_value=1  i_L_nominal_unit=A
  Mechanical Rotational Reference : fl_lib/Mechanical/Rotational Elements/Mechanical Rotational Reference
  PS-Simulink Converter : nesl_utility/PS-Simulink Converter  PhysicalDomain=network_engine_domain  SubClassName=ps_output  LeftPortType=input  RightPortType=output  PseudoPeriodic=off  Frequencies=[]  VectorFormat=1-D array  Unit=inherit  AffineConversion=off
  PS-Simulink Converter3 : nesl_utility/PS-Simulink Converter  PhysicalDomain=network_engine_domain  SubClassName=ps_output  LeftPortType=input  RightPortType=output  PseudoPeriodic=off  Frequencies=[]  VectorFormat=1-D array  Unit=inherit  AffineConversion=off
  Power Measurement (Three-Phase) : eePowerMeasurement/Power Measurement (Three-Phase)  LabelModeActiveChoice=Discrete  F=60  K=[0 1 2 3]  Seq=Positive  Ts=Ts
  RLC (Three-Phase) : ee_lib/Passive/RLC Assemblies/RLC (Three-Phase)  port_option=ee.enum.threePhasePort.composite  component_structure=2  R=1 Ohm  L=5e-4 H  C=1e-6 F  R_parasitic=1e-6 Ohm  G_parasitic=1e-6 1/Ohm  IL_specify=on  IL_priority=High  IL=[0, 0, 0] A  IL_nominal_specify=off  IL_nominal_value=1  IL_nominal_unit=A  VC_specify=on  VC_priority=High  VC=[0, 0, 0] V  VC_nominal_specify=off  VC_nominal_value=1  VC_nominal_unit=V
      settings: InternalSimscapePortConfiguration="{\"Bottom\":[],\"Left\":[{\"id\":\"N1\",\"label\":\"~1\",\"type\":\"foundation.electrical.three_phase\"}],\"Right\":[{\"id\":\"N2\",\"label\":\"~2\",\"type\":\"foundation.electrical.three_phase\"}],\"Top\":[]}"
  Sensing current : Subsystem
      mask Display: disp('i')
  Sensing voltage : Subsystem
  Simulink-PS Converter : nesl_utility/Simulink-PS Converter  PhysicalDomain=network_engine_domain  SubClassName=ps_input  LeftPortType=input  RightPortType=output  PseudoPeriodic=off  Frequencies=[]  NoiseDistribution=none  NoiseParameters=[]  Unit=rad/s  AffineConversion=off  FilteringAndDerivatives=provide  SimscapeFilterOrder=1  InputFilterTimeConstant=0.001  UdotUserProvided=0
  Sum : Sum  Inputs=|+-
  Sum1 : Sum  Inputs=|-+
  Synchronous Machine Salient Pole : ee_lib/Electromechanical/Synchronous/Synchronous Machine Salient Pole  port_option=ee.enum.threePhasePort.composite  SRated=45e6 V*A  VRated=9.8e3 V  FRated=240 Hz  nPolePairs=4  param_option=ee.enum.sm.parameterization.standard  fieldCircuitParameterization_option=ee.enum.sm.fieldparameterization.current  baseEfd=216.54 V  baseIfd=200 A  zero_sequence=ee.enum.park.zerosequence.exclude  axes_param=ee.enum.rotorangle.daxis  Ladu=0.9  Laqu=0.55  L0=0.15  Ll=0.15  Ra=0.006  Lfd=0.2571  Rfd=0.0006  L1d=0.2  R1d=0.0354  L1q=0.2567  R1q=0.0428  Xl=0.08  Xd=1.352  Xq=0.836  X0=0.15  Xdd=0.296  Xddd=0.148  Xqdd=0.122  d_option=ee.enum.circuit.open  Td0d=4.141 s  Tdd=1.75 s  Td0dd=0.027 s  Tddd=0.0214 s  q_option=ee.enum.circuit.open  Tq0dd=0.184 s  Tqdd=0.0232 s  saturation_option=ee.enum.saturation.exclude  saturation_ifd=[0, .48, .76, 1.38, 1.79]  saturation_Vag=[0, .43, .59, .71, .76]  initialization_option=ee.enum.sm.initialization.electrical  source_type=ee.enum.sm.load_flow_source_type.Swing  Vmag0=13.8e3 V  Vang0=0 deg  Pt0=1e6 V*A  Qt0=0 V*A  minimum_pu=0.95  phase_search_range=[-30, 30] deg  gmin=1e-6 S  connection_option=ee.enum.Connection.wye  num_q_dampers=1  rotor_offset=-pi / 2 rad  pu_psid_specify=off  pu_psid_priority=None  pu_psid=0  pu_psid_nominal_specify=off  pu_psid_nominal_value=1  pu_psid_nominal_unit=1  pu_psiq_specify=off  pu_psiq_priority=None  pu_psiq=0  pu_psiq_nominal_specify=off  pu_psiq_nominal_value=1  pu_psiq_nominal_unit=1  pu_psifd_specify=off  pu_psifd_priority=None  pu_psifd=0  pu_psifd_nominal_specify=off  pu_psifd_nominal_value=1  pu_psifd_nominal_unit=1  pu_psi1d_specify=off  pu_psi1d_priority=None  pu_psi1d=0  pu_psi1d_nominal_specify=off  pu_psi1d_nominal_value=1  pu_psi1d_nominal_unit=1  pu_psi1q_specify=off  pu_psi1q_priority=None  pu_psi1q=0  pu_psi1q_nominal_specify=off  pu_psi1q_nominal_value=1  pu_psi1q_nominal_unit=1  angular_position_diff_specify=off  angular_position_diff_priority=None  angular_position_diff=18 deg  angular_position_diff_nominal_specify=off  angular_position_diff_nominal_value=1  angular_position_diff_nominal_unit=deg  Tmeas=298.15 K  alpha=3.93e-3 1/K  stator_thermal_mass=100 J/K  rotor_thermal_mass=200 J/K  temperatureA_specify=off  temperatureA_priority=High  temperatureA=25 degC  temperatureA_nominal_specify=off  temperatureA_nominal_value=1  temperatureA_nominal_unit=degC  temperatureB_specify=off  temperatureB_priority=High  temperatureB=25 degC  temperatureB_nominal_specify=off  temperatureB_nominal_value=1  temperatureB_nominal_unit=degC  temperatureC_specify=off  temperatureC_priority=High  temperatureC=25 degC  temperatureC_nominal_specify=off  temperatureC_nominal_value=1  temperatureC_nominal_unit=degC  temperatureR_specify=off  temperatureR_priority=High  temperatureR=25 degC  temperatureR_nominal_specify=off  temperatureR_nominal_value=1  temperatureR_nominal_unit=degC
      settings: InternalSimscapePortConfiguration="{\"Bottom\":[],\"Left\":[{\"id\":\"fd_p\",\"label\":\"fd+\",\"type\":\"foundation.electrical.electrical\"},{\"id\":\"fd_n\",\"label\":\"fd-\",\"type\":\"foundation.electrical.electrical\"},{\"id\":\"R\",\"label\":\"R\",\"type\":\"foundation.mechanical.rotational.rotational\"},{\"id\":\"C\",\"label\":\"C\",\"type\":\"foundation.mechanical.rotational.rotational\"}],\"Right\":[{\"id\":\"pu_output\",\"label\":\"pu\",\"type\":\"output\"},{\"id\":\"N\",\"label\":\"~\",\"type\":\"foundation.electrical.three_phase\"}],\"Top\":[]}"
  Terminator{,1..5} (6 alike) : Terminator
  Three-phase PLL : eeSinusoidalMeasurement/Sinusoidal Measurement (PLL, Three-Phase)  Kp_LF=45  Ki_LF=1250  F0=60  Theta0=0  Ts=TsELEC
  Thyristor converter : ee_lib/Semiconductors & Converters/Converters/Converter (Three-Phase)  port_option=ee.enum.threePhasePort.composite  fidelity_option=ee.enum.converters.fidelity.detailed  device_type=ee.enum.converters.switchingdevice.thyristor  showThermalPort=false  K=0  Vth=6 V  Vgt=.5 V  Vgt_off=-1 V  Ih=1 A  Vf=0.8 V  Ron=0.001 Ohm  Rds=0.001 Ohm  Goff=1e-5 1/Ohm  Eon_scalar=22.86e-3 J  Eoff_scalar=17.14e-3 J  Eoff_natural_commutation=10e-3 J  Voff=300 V  Iout_scalar=600 A  onCurrentMeasDelay=0 s  useCurrentFromPreviousCycle=false  useVoltageFromPreviousCycle=false  diode_param=ee.enum.converters.protectiondiode.none  diode_Vf=0.8 V  diode_Ron=0.001 Ohm  diode_Goff=1e-5 1/Ohm  diode_C=50 nF  diode_iRM=-235 A  diode_iF=300 A  diode_idot=-50 A/us  diode_trr_param=ee.enum.converters.diodetrr.trr_factor  diode_trr_factor=3  diode_trr=15 us  diode_Qrr=1.5e+3 s*uA  diode_rec_loss_model=ee.enum.diode.reverseRecoveryModel.fixed  diode_ErecVal=0 J  diode_scaleWithIandV=false  diode_ErecMat=zeros(2, 3) J  diode_TjrecVec=[298.15, 398.15] K  diode_IfrecVec=[.1, 1, 10] A  diode_IrecVal=10 A  diode_VrecVal=10 V  diode_tFilter=1 / 1000 / 100 s  thermal_network_parameterization=ee.enum.thermalNetworkTopology.external  Rth=[.08, .5] K/W  Rth_Cauer=[.08, .1, .5] K/W  Rth_Foster=[.08, .14, .22, .16] K/W  thermal_mass_parameterization=ee.enum.thermalNetwork.timeconstant  thermal_mass=[.01, .5] J/K  thermal_mass_Cauer=[.01, .1, .5] J/K  thermal_mass_Foster=[.001, .005, .05, .5] J/K  thermal_time_constant=[.001, .2] s  thermal_time_constant_Cauer=[.001, .1, .2] s  thermal_time_constant_Foster=[7e-05, .0007, .01, .08] s  thermal_mass_initial_temperatures=[25, 25] degC  thermal_mass_initial_temperatures_Cauer=[25, 25, 25] degC  junction_thermal_mass=0.01 J/K  Tvec_initial_Foster=[25, 25, 25, 25] degC  snubber_type=ee.enum.converters.snubber.exclude  Cs=1e-7 F  Rs=0.1 Ohm  Vce_loss=[0, 150, 300] V
  Unit Delay : UnitDelay  SampleTime=TsELEC  HasFrameUpgradeWarning=on
  Unit Delay1 : UnitDelay  SampleTime=-1  HasFrameUpgradeWarning=on
  Voltage Sensor : fl_lib/Electrical/Electrical Sensors/Voltage Sensor
  Wye-Connected Load : ee_lib/Passive/RLC Assemblies/Wye-Connected Load  port_option=ee.enum.threePhasePort.composite  parameterization=2  component_structure=1  component_structure_PQ=1  R=1 Ohm  L=1e-3 H  C=1e-6 F  VRated=9.8e3 V  FRated=60 Hz  P=1.8e6 W  Qpos=1e2 V*A  Qneg=-1e2 V*A  R_parasitic=1e-6 Ohm  G_parasitic=1e-6 1/Ohm  R_parasitic_PQ=1e-6 Ohm  G_parasitic_PQ=1e-6 1/Ohm  Vmag0=24e3 V  Vang0=0 deg  Freq0=60 Hz  IL_specify=on  IL_priority=High  IL=[0, 0, 0] A  IL_nominal_specify=off  IL_nominal_value=1  IL_nominal_unit=A  VC_specify=on  VC_priority=High  VC=[0, 0, 0] V  VC_nominal_specify=off  VC_nominal_value=1  VC_nominal_unit=V
  + : PMIOPort  Side=Right
  - : PMIOPort  Port=2  Side=Right
  Vt_Ifd : Outport
  wires:
  [Iabc1] -> Power Measurement (Three-Phase)/2  "Iabc1"
  [Vabc1] -> Power Measurement (Three-Phase)/1  "Vabc1"
  PS-Simulink Converter3/1 -> Terminator/1  "Tm1"
  Constant/1 -> Simulink-PS Converter/1
  Unit Delay/1 -> 6-pulse generator/1
  Gain/1 -> Three-phase PLL/1
  Three-phase PLL/2 -> Unit Delay/1
  [Vabc1] -> Gain/1  "Vabc"
  6-pulse generator/1 -> Gate driver/1(S)
  Discrete-Time Integrator1/1 -> 6-pulse generator/2  "alpha1"
  Three-phase PLL/3 -> Terminator1/1
  Three-phase PLL/1 -> Terminator2/1
  Unit Delay1/1 -> Vt_Ifd/1
  " field circuit"/1(Vt_Ifd) -> Unit Delay1/1
  [Z1_Efd] -> " field circuit"/1(Efd_pu)  "Efd1"
  Power Measurement (Three-Phase)/1 -> Terminator3/1  "P1"
  Power Measurement (Three-Phase)/2 -> Terminator4/1  "Q1"
  PS-Simulink Converter/1 -> Sum/1
  Sum/1 -> Discrete-Time Integrator/1
  Discrete-Time Integrator/1 -> Terminator5/1, Sum1/2, Sum/2  "VDC_PGM1"
  Sum1/1 -> Discrete-Time Integrator1/1
  Constant1/1 -> Sum1/1
  connections:
  Electrical Reference1/LConn1 -- Wye-Connected Load/RConn1
  PS-Simulink Converter3/LConn1 -- Ideal Torque Sensor/RConn2
  Ideal Torque Sensor/RConn1 -- Ideal Angular Velocity Source/LConn1
  Simulink-PS Converter/RConn1 -- Ideal Angular Velocity Source/RConn1
  Synchronous Machine Salient Pole/LConn4 -- Mechanical Rotational Reference/LConn1 -- Ideal Angular Velocity Source/RConn2
  Synchronous Machine Salient Pole/LConn3 -- Ideal Torque Sensor/LConn1
  Sensing voltage/RConn1 -- Grounded Neutral2/LConn1
  Thyristor converter/LConn2 -- Sensing current/RConn1
  Gate driver/RConn1 -- Thyristor converter/LConn1
  Synchronous Machine Salient Pole/LConn1 -- " field circuit"/RConn1
  " field circuit"/LConn1 -- Synchronous Machine Salient Pole/RConn1
  " field circuit"/RConn2 -- Synchronous Machine Salient Pole/LConn2
  Thyristor converter/RConn2 -- Capacitor1/LConn1 -- Inductor/LConn1 -- Voltage Sensor/LConn1
  PS-Simulink Converter/LConn1 -- Voltage Sensor/RConn1
  Inductor/RConn1 -- +/RConn1
  Thyristor converter/RConn1 -- Inductor1/LConn1 -- Capacitor1/RConn1 -- Voltage Sensor/RConn2
  RLC (Three-Phase)/RConn1 -- Sensing current/LConn1
  Wye-Connected Load/LConn1 -- Sensing voltage/LConn1 -- RLC (Three-Phase)/LConn1 -- Synchronous Machine Salient Pole/RConn2
  Inductor1/RConn1 -- -/RConn1
